simulink model "dynamic_model_tab"  (R2022b)
settings: Solver=VariableStepAuto  StartTime=0.0  StopTime=30e-2  RelTol=1e-3
undefined symbols (not defined in the file): Ion, Lithium
libraries: spsMosfetLib x12, spsMeanLib x8, eeGeneralControl x7, spsSeriesRLCBranchLib x6, spsCurrentMeasurementLib x4, spsMultimeterLib x3, slpidlib x3, hdlsllib x2, simulink x2, spsDiscreteVariableTimeDelayLib x2, spsEdgeDetectorLib x2, spsBatteryLib x1
settings Model: Creator=srikr  LastModifiedBy=srikri

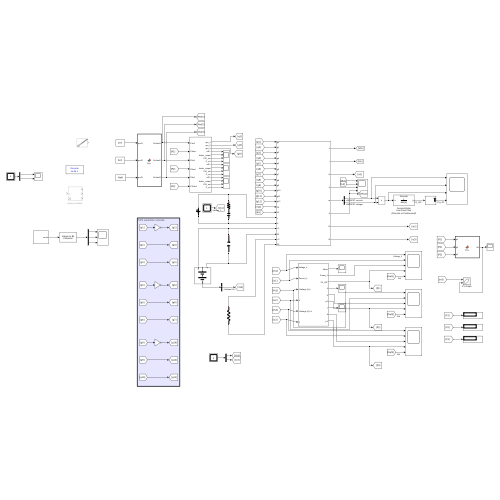
[thumbnail: Simulink's stored preview of the top-level diagram]
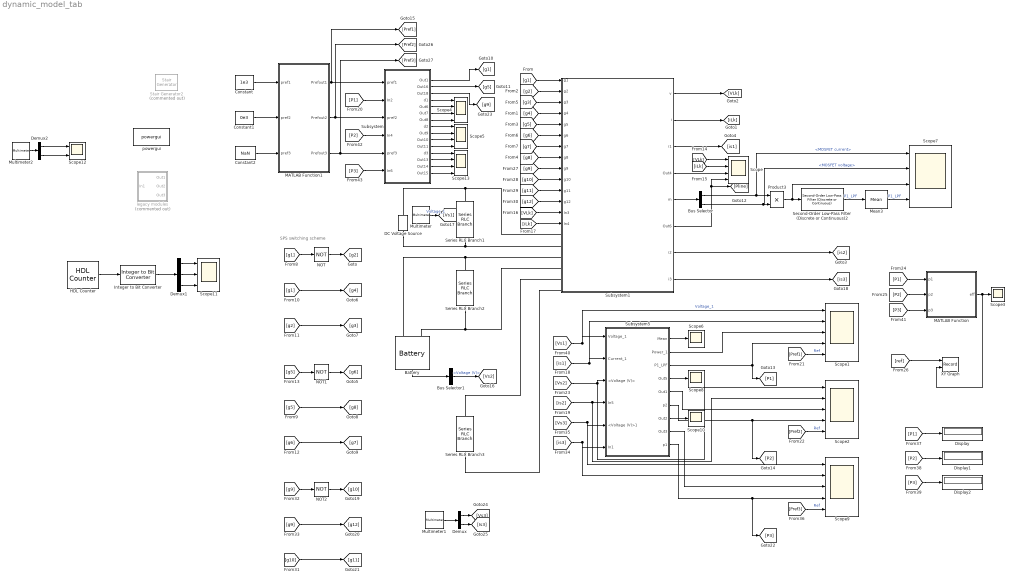
== system dynamic_model_tab ==
  note: SPS switching scheme
  Battery : spsBatteryLib/Battery  BatType=Lithium-Ion  ShowTempParam=off  ThermalPreset=no  ShowAgeParam=off  NomV=96  NomQ=150  SOC=100  Batt_Tr=30  PresetModel=on  MaxQ=150  MinV=72  FullV=111.7428  Dis_rate=65.2174  R=0.0064  Normal_OP=135.6522  expZone="[103.717      7.369565]"  current=[6.5 13 32.5]  Units=Time  Tci=20  NomT=20  T2=-30  MaxQ2=4.8  FullV2=7.1  Normal_OP2=5.655  expZone2="[6.58           1]"  Rca=0.6  ti=2000  Dp=0  Neq0=0  Tsim=1e6  Ta1=25  Qeol=5.4*0.9  Reol=0.013333*1.2  Char_age=[2.3478, 3]  Dis_age=[2.3478, 10]  N1=1500  N2=10500  N3=1000  N4=1400  Ta2=45  N5=950
  Bus Selector : BusSelector  OutputSignals=MOSFET current,MOSFET voltage
  Bus Selector1 : BusSelector  OutputSignals=Voltage (V)
  Constant : Constant  Value=1e3
  Constant1 : Constant  Value=0e3
  Constant2 : Constant  Value=NaN
  DC Voltage Source : spsDCVoltageSourceLib/DC Voltage Source  Amplitude=120  Measurements=Voltage
  Demux : Demux  Outputs=2
  Demux1 : Demux  Outputs=3
  Demux2 : Demux  Outputs=2
  Display : Display
  Display1 : Display
  Display2 : Display
  HDL Counter : hdlsllib/Sources/HDL Counter  CountType=Modulo  CountInit=0  CountStep=1  CountMax=7  CountFromType=Initial value  CountFrom=0  CountResetPort=off  CountLoadPort=off  CountEnbPort=off  CountDirPort=off  CountHitOutputPort=off  CountDataType=Unsigned  CountWordLen=8  CountFracLen=0  CountSampTime=1e-3
  Integer to Bit Converter : simulink/Logic and Bit Operations/Integer to Bit Converter  nbits=3  signedInputValues=Unsigned  bitOrder=MSB first  outDtype=Inherit via internal rule
  MATLAB Function : MATLAB Function  TreatAsAtomicUnit=on
  MATLAB Function1 : MATLAB Function  TreatAsAtomicUnit=on
  Mean3 : spsMeanLib/Mean  Freq=50e3  Vinit=0  Ts=0
  Multimeter : spsMultimeterLib/Multimeter  L=12  sel=5  yselected={}  Gain=1  OutputType=Complex  PlotAtSimulationStop=off  PhasorSimulation=off
  Multimeter1 : spsMultimeterLib/Multimeter  L=12  sel=[1 3]  yselected={}  Gain=[1 1]  OutputType=Complex  PlotAtSimulationStop=off  PhasorSimulation=off
  Multimeter2 : spsMultimeterLib/Multimeter  L=12  sel=[2 7]  yselected={}  Gain=[1 1]  OutputType=Complex  PlotAtSimulationStop=off  PhasorSimulation=off
  NOT : Logic  Operator=NOT  IconShape=distinctive  AllPortsSameDT=off  OutDataTypeStr=boolean
  NOT1 : Logic  Operator=NOT  IconShape=distinctive  AllPortsSameDT=off  OutDataTypeStr=boolean
  NOT2 : Logic  Operator=NOT  IconShape=distinctive  AllPortsSameDT=off  OutDataTypeStr=boolean
  Product3 : Product
  Scope{,4..5,7,13} (5 alike) : Scope  NumInputPorts=4
  Scope1 : Scope  NumInputPorts=5
  Scope{3,6,8,10} (4 alike) : Scope
  Scope11 : Scope  NumInputPorts=3
  Scope12 : Scope  NumInputPorts=2
  Scope2 : Scope  NumInputPorts=5
  Scope9 : Scope  NumInputPorts=5
  Second-Order Low-Pass Filter (Discrete or Continuous)2 : eeGeneralControl/Second-Order Low-Pass Filter (Discrete or Continuous)  A1=2*sqrt(2)*1e-3  A2=(1e-3)^2  init_option=Inherited from block input  x0=0  Ts=-1
      settings: LibrarySourceBlock=|
      | ee_sl_lib/General Control/Second-Order
      | Low-Pass Filter
      | (Discrete or Continuous)
  Series RLC Branch1 : spsSeriesRLCBranchLib/Series RLC Branch  LConnTagsString=__new0  RConnTagsString=__new0  BranchType=RC  Resistance=1e-9  Inductance=1e-3  SetiL0=off  InitialCurrent=0  Capacitance=1000e-6  Setx0=off  InitialVoltage=0  Measurements=None
  Series RLC Branch2 : spsSeriesRLCBranchLib/Series RLC Branch  LConnTagsString=__new0  RConnTagsString=__new0  BranchType=C  Resistance=1e-9  Inductance=1e-3  SetiL0=off  InitialCurrent=0  Capacitance=1000e-6  Setx0=off  InitialVoltage=0  Measurements=None
  Series RLC Branch3 : spsSeriesRLCBranchLib/Series RLC Branch  LConnTagsString=__new0  RConnTagsString=__new0  BranchType=R  Resistance=(380^2) / (7.5e3)  Inductance=1e-3  SetiL0=off  InitialCurrent=0  Capacitance=1000e-6  Setx0=off  InitialVoltage=0  Measurements=Branch voltage and current
  Stair Generator2 : spsStairGeneratorLib/Stair Generator  Commented=on  t=[0:0.025:1]*100e-2*(1-0.1)  e=([-1:0.05:1])*2.8e3  Ts=0
  Subsystem : Subsystem
  Subsystem1 : Subsystem
  Subsystem5 : Subsystem
  XY Graph : Record  FileSettingsInternal="{\"entries\":[{\"content\":{\"excelSettings\":{\"content\":{},\"type\":\"Streamout.ExcelSettings\"}},\"type\":\"Streamout.FileSettingStorage\",\"uuid\":\"f45d7055-9ecb-48ab-a96f-031432f1a6f8\"}],\"packageUris\":[\"http://schema.mathworks.com/mf0/streamout_blocks/R2020a\"],\"version\":\"1.0\"}"  Layout=[1 1]  SignalsInternal="{\"entries\":[{\"content\":{\"signals\":[{\"content\":{\"blockPath\":[\"dynamic_model_tab/XY Graph\"],\"channel\":[],\"dimensions\":[1],\"domain\":\"dynamic_model_tab/XY Graph\",\"lineColor\":\"#7e2f8e\",\"plots\":[],\"port\":1,\"sid\":[],\"signalID\":33,\"signalName\":\"From26\"},\"type\":\"RecordBlkView.Signal\",\"uuid\":\"0354a216-3750-4216-9fc3-88f8f814a368\"},{\"content\":{\"blockPath\":[\"dynamic_model_tab/XY Graph\"],\"channel\":[],\"dimensions\":[1],\"domain\":\"dynamic_model_tab/XY Graph\",\"lineColor\":\"#ff13a6\",\"plots\":[],\"port\":2,\"sid\":[],\"signalID\":36,\"signalName\":\"MATLAB Function\"},\"type\":\"RecordBlkView.Signal\",\"uuid\":\"1e314882-d803-43e1-8662-509fc0bc40a2\"}]},\"type\":\"RecordBlkView.InputSignals\",\"uuid\":\"ae186877-b2c7-4f81-851d-3e3b29c6325c\"}],\"packageUris\":[\"http://schema.mathworks.com/mf0/streamout_blocks/R2020a\"],\"version\":\"1.0\"}"  VisualizationBindings="{\"xyplotplugin\":{\"info\":[{\"series\":[],\"subplotID\":1}]}}"  CompatibilityTag=XY
  legacy modules : Subsystem  Commented=on
  powergui : spspowerguiLib/powergui  Priority=1  SimulationMode=Discrete  SampleTime=1e-6  frequency=60  Iterations=50  frequencyindice=0  Pbase=100e6  ErrMax=1e-4  UnitsV=kV  UnitsW=MW  buscounter=0  FunctionMessages=off  echomessages=off  EnableUseOfTLC=off  CurrentSourceSwitches=off  DisableSnubberDevices=off  DisableRonSwitches=off  DisableVfSwitches=off  DisplayEquations=off  AutomaticDiscreteSolvers=off  SolverType=Tustin/Backward Euler (TBE)  Interpol=off  ExternalGateDelay=off  methode=off  Ts=100  x0status=blocks  SPID=on  SwTol=0  HookPort=off  NonlinearTolerance=1e-4  nMaxIteration=100  ContinueOnMaxIteration=off  RestoreLinks=warning  ResistiveCurrentMeasurement=off  Frange=[0:2:500]  Ylog=off  Xlog=on  ShowGrid=off  save=off  variable=ZData  structure=0  ZoomFFT=off  StartTime=0.0  cycles=1  DisplayStyle=1  fundamental=60  FreqAxis=off  MaxFrequency=1000  frequencyindicesteady=1  RmsSteady=1  display=off
  wires:
  [VLk] -> Scope/1
  [iLk] -> Scope/2
  [Vs1] -> Scope1/1, Subsystem5/1(Voltage_1)  "Voltage_1"
  [is2] -> Subsystem5/4(In5), Scope2/2
  Bus Selector/1 -> Scope7/1, Product3/1  "<MOSFET current>"
  Bus Selector/2 -> Scope7/2, Product3/2  "<MOSFET voltage>"
  Product3/1 -> Scope7/3, Second-Order Low-Pass Filter (Discrete or Continuous)2/1
  [Pref1] -> Scope1/5  "Ref"
  Battery/1 -> Bus Selector1/1
  [P1] -> Subsystem/2(In2)
  Subsystem/1(Out1) -> [g1]
  Subsystem/2(Out16) -> [g5]
  Subsystem/4(d1) -> Scope4/1
  Subsystem/5(Out6) -> Scope4/2
  Subsystem/6(Out7) -> Scope4/3
  Subsystem/7(Out8) -> Scope4/4
  Subsystem5/1(Mean) -> Scope6/1
  Subsystem5/2(Power_1) -> Scope1/3
  Subsystem1/6(Out6) -> [Pline], Scope/4
  [g4] -> Subsystem1/4(g4)
  [g2] -> Subsystem1/2(g2)
  [VLk] -> Subsystem1/13(In3)
  [iLk] -> Subsystem1/14(In4)
  [g1] -> Subsystem1/1(g1)
  [g3] -> Subsystem1/3(g3)
  [g5] -> Subsystem1/5(g5)
  [g7] -> Subsystem1/7(g7)
  [g6] -> Subsystem1/6(g6)
  [g8] -> Subsystem1/8(g8)
  Subsystem1/1(v) -> [VLk]
  Subsystem1/2(i) -> [iLk]
  Subsystem1/3(i1) -> [is1]
  Subsystem1/4(Out4) -> Scope/3
  Subsystem1/5(m) -> Bus Selector/1
  Subsystem1/7(i2) -> [is2]
  [g1] -> NOT/1
  NOT/1 -> [g2]
  [g5] -> [g8]
  NOT1/1 -> [g6]
  [g6] -> [g7]
  [g5] -> NOT1/1
  [g2] -> [g3]
  [g1] -> [g4]
  Subsystem5/5(Out1) -> Scope2/3
  [is1] -> Scope1/2, Subsystem5/2(Current_1)
  [Pref2] -> Scope2/5  "Ref"
  Bus Selector1/1 -> [Vs2]  "<Voltage (V)>"
  [Vs2] -> Subsystem5/3(<Voltage (V)>), Scope2/1
  Second-Order Low-Pass Filter (Discrete or Continuous)2/1 -> Mean3/1  "P1_LPF"
  Mean3/1 -> Scope7/4  "P1_LPF"
  Subsystem5/3(P1_LPF) -> [P1], Scope1/4
  MATLAB Function/1(eff) -> XY Graph/2, Scope3/1
  Subsystem5/4(Out5) -> Scope8/1
  Subsystem5/6(p2) -> [P2], Scope2/4
  [P1] -> MATLAB Function/1(p1)
  [P2] -> MATLAB Function/2(p2)
  [ref] -> XY Graph/1
  [g9] -> Subsystem1/9(g9)
  [g10] -> Subsystem1/10(g10)
  [g11] -> Subsystem1/11(g11)
  [g12] -> Subsystem1/12(g12)
  Subsystem1/8(i3) -> [is3]
  [g9] -> [g12]
  [g9] -> NOT2/1
  [g10] -> [g11]
  NOT2/1 -> [g10]
  [Vs3] -> Scope9/1, Subsystem5/5(<Voltage (V)>1)
  [Pref3] -> Scope9/5  "Ref"
  [is3] -> Scope9/2, Subsystem5/6(In1)
  Subsystem5/9(p1) -> [P3], Scope9/4
  Subsystem5/8(Out3) -> Scope9/3
  Subsystem5/7(Out2) -> Scope10/1
  Subsystem/3(Out18) -> [g9]
  [P1] -> Display/1
  [P2] -> Display1/1
  [P3] -> Display2/1
  Multimeter/1 -> [Vs1]  "Voltage_1"
  Multimeter1/1 -> Demux/1
  Demux/1 -> [Vs3]
  Demux/2 -> [Is3]
  Integer to Bit Converter/1 -> Demux1/1
  HDL Counter/1 -> Integer to Bit Converter/1
  Demux1/1 -> Scope11/1
  Demux1/2 -> Scope11/2
  Demux1/3 -> Scope11/3
  Multimeter2/1 -> Demux2/1
  Demux2/1 -> Scope12/1
  Demux2/2 -> Scope12/2
  [P3] -> MATLAB Function/3(p3)
  Subsystem/11(Out11) -> Scope5/4
  Subsystem/9(Out9) -> Scope5/2
  Subsystem/8(d2) -> Scope5/1
  Subsystem/10(Out10) -> Scope5/3
  Subsystem/15(Out15) -> Scope13/4
  Subsystem/13(Out13) -> Scope13/2
  Subsystem/12(d3) -> Scope13/1
  Subsystem/14(Out14) -> Scope13/3
  [P2] -> Subsystem/4(In4)
  [P3] -> Subsystem/6(In6)
  Constant/1 -> MATLAB Function1/1(pref1)
  Constant1/1 -> MATLAB Function1/2(pref2)
  Constant2/1 -> MATLAB Function1/3(pref3)
  MATLAB Function1/1(Prefout1) -> Subsystem/1(pref1), [Pref1]
  MATLAB Function1/2(Prefout2) -> Subsystem/3(pref2), [Pref2]
  MATLAB Function1/3(Prefout3) -> Subsystem/5(pref3), [Pref3]
  connections:
  Series RLC Branch1/RConn1 -- DC Voltage Source/LConn1 -- Subsystem1/LConn2
  Series RLC Branch2/RConn1 -- Subsystem1/LConn4 -- Battery/LConn2
  Series RLC Branch2/LConn1 -- Subsystem1/LConn3 -- Battery/LConn1
  Subsystem1/LConn1 -- DC Voltage Source/RConn1 -- Series RLC Branch1/LConn1
  Series RLC Branch3/RConn1 -- Subsystem1/LConn6
  Series RLC Branch3/LConn1 -- Subsystem1/LConn5

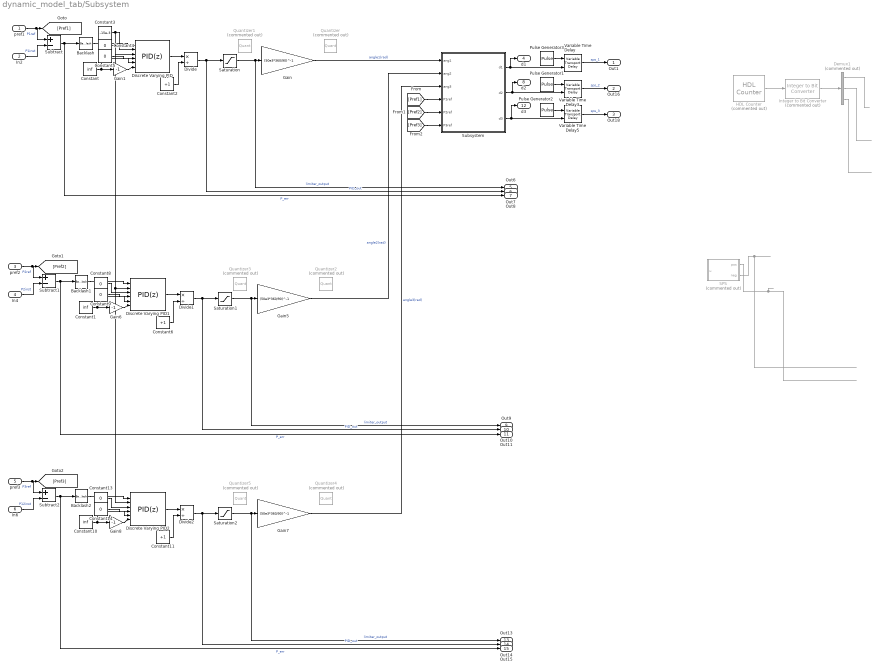
== system dynamic_model_tab/Subsystem ==
  pref1 : Inport
  In2 : Inport  Port=2
  pref2 : Inport  Port=3
  In4 : Inport  Port=4
  pref3 : Inport  Port=5
  In6 : Inport  Port=6
  Backlash : Backlash  BacklashWidth=0
  Backlash1 : Backlash  BacklashWidth=0
  Backlash2 : Backlash  BacklashWidth=0
  Constant : Constant  Value=inf
  Constant1 : Constant  Value=inf
  Constant10 : Constant  Value=inf
  Constant11 : Constant  Value=+1
  Constant{4..5,8..9,13..14} (6 alike) : Constant  Value=0
  Constant2 : Constant  Value=+1
  Constant3 : Constant  Value=-15e-3
  Constant6 : Constant  Value=+1
  Demux1 : Demux  Commented=on  Outputs=3
  Discrete Varying PID : slpidlib/PID Controller  Controller=PID  Form=Parallel  TimeDomain=Discrete-time  UseExternalTs=off  SampleTime=-1  IntegratorMethod=Forward Euler  FilterMethod=Forward Euler  ControllerParametersSource=external  P=1  I=1  UseKiTs=off  D=0  N=100  UseFilter=off  TunerSelectOption=Transfer Function Based (PID Tuner App)  InitialConditionSource=internal  InitialConditionForIntegrator=0  InitialConditionForFilter=0  DifferentiatorICPrevScaledInput=0  ExternalReset=none  TrackingMode=off  Kt=1  LimitOutput=on  SatLimitsSource=external  UpperSaturationLimit=inf  LowerSaturationLimit=-inf  LinearizeAsGain=on  AntiWindupMode=none  Kb=1  LimitIntegrator=off  UpperIntegratorSaturationLimit=inf  LowerIntegratorSaturationLimit=-inf  POutMin=[]  POutMax=[]  IOutMin=[]  IOutMax=[]  DOutMin=[]  DOutMax=[]  NOutMin=[]  NOutMax=[]  SumOutMin=[]  SumOutMax=[]  SaturationOutMin=[]  SaturationOutMax=[]  PParamMin=[]  PParamMax=[]  IParamMin=[]  IParamMax=[]  DParamMin=[]  DParamMax=[]  NParamMin=[]  NParamMax=[]  KbParamMin=[]  KbParamMax=[]  KtParamMin=[]  KtParamMax=[]  KbOutMin=[]  KbOutMax=[]  KtOutMin=[]  KtOutMax=[]  IntegratorOutMin=[]  IntegratorOutMax=[]  FilterOutMin=[]  FilterOutMax=[]  SumI1OutMin=[]  SumI1OutMax=[]  SumI2OutMin=[]  SumI2OutMax=[]  SumI3OutMin=[]  SumI3OutMax=[]  SumI4OutMin=[]  SumI4OutMax=[]  SumDOutMin=[]  SumDOutMax=[]  DifferentiatorOutMin=[]  DifferentiatorOutMax=[]  FilterDiffOutCoefMin=[]  FilterDiffOutCoefMax=[]  ReciprocalOutMin=[]  ReciprocalOutMax=[]  SumDenOutMin=[]  SumDenOutMax=[]  SumNumOutMin=[]  SumNumOutMax=[]  DivideOutMin=[]  DivideOutMax=[]  UdiffTsProdOutMin=[]  UdiffTsProdOutMax=[]  NTsProdOutMin=[]  NTsProdOutMax=[]  UintegralTsProdOutMin=[]  UintegralTsProdOutMax=[]  UngainTsProdOutMin=[]  UngainTsProdOutMax=[]  ClampingZeroOutDataTypeStr=Inherit: Inherit via back propagation  ClampingZeroOutMin=[]  ClampingZeroOutMax=[]  FilterDenConstantOutDataTypeStr=Inherit: Inherit via back propagation  FilterDenConstantOutMin=[]  FilterDenConstantOutMax=[]  PCopyOutDataTypeStr=Inherit: Inherit via back propagation  PCopyOutMin=[]  PCopyOutMax=[]  NCopyOutDataTypeStr=Inherit: Inherit via back propagation  NCopyOutMin=[]  NCopyOutMax=[]  IntegratorContinuousStateAttributes=''  IntegratorStateMustResolveToSignalObject=off  IntegratorRTWStateStorageClass=Auto  FilterContinuousStateAttributes=''  FilterStateMustResolveToSignalObject=off  FilterRTWStateStorageClass=Auto  ParallelPVariant=ExternalParameters  IdealPVariant=Disabled  IVariant=ExternalParameters  DVariant=ExternalParameters  IntegratorVariant=Discrete  SatVariant=External  AWVariant=Passthrough  PCopyVariant=Disabled  TRVariant=Disabled  FdbkBlocksVariant=Forward  IdealPFdbkVariant=Disabled  SatFdbkVariant=Disabled  DerivativeFilterVariant=Differentiator  NVariant=Passthrough  NCopyVariant=Disabled_SignalSpec  FilterICVariant=InternalICsDifferentiator  IntegratorICVariant=InternalICs  ExternalResetVariant=Disabled  TRSumVariant=Passthrough  SumFdbkVariant=Disabled  SumVariant=Sum_PID  TsampFilterVariant=InternalTs  TsampNgainVariant=Passthrough  TsampIntegralVariant=Passthrough  ExternalSaturationOutDataTypeStr=Inherit: Same as second input
      settings: LibrarySourceBlock=cstblocks/Linear Parameter Varying/Discrete Varying PID
  Discrete Varying PID1 : slpidlib/PID Controller  Controller=PID  Form=Parallel  TimeDomain=Discrete-time  UseExternalTs=off  SampleTime=-1  IntegratorMethod=Forward Euler  FilterMethod=Forward Euler  ControllerParametersSource=external  P=1  I=1  UseKiTs=off  D=0  N=100  UseFilter=off  TunerSelectOption=Transfer Function Based (PID Tuner App)  InitialConditionSource=internal  InitialConditionForIntegrator=0  InitialConditionForFilter=0  DifferentiatorICPrevScaledInput=0  ExternalReset=none  TrackingMode=off  Kt=1  LimitOutput=on  SatLimitsSource=external  UpperSaturationLimit=inf  LowerSaturationLimit=-inf  LinearizeAsGain=on  AntiWindupMode=none  Kb=1  LimitIntegrator=off  UpperIntegratorSaturationLimit=inf  LowerIntegratorSaturationLimit=-inf  POutMin=[]  POutMax=[]  IOutMin=[]  IOutMax=[]  DOutMin=[]  DOutMax=[]  NOutMin=[]  NOutMax=[]  SumOutMin=[]  SumOutMax=[]  SaturationOutMin=[]  SaturationOutMax=[]  PParamMin=[]  PParamMax=[]  IParamMin=[]  IParamMax=[]  DParamMin=[]  DParamMax=[]  NParamMin=[]  NParamMax=[]  KbParamMin=[]  KbParamMax=[]  KtParamMin=[]  KtParamMax=[]  KbOutMin=[]  KbOutMax=[]  KtOutMin=[]  KtOutMax=[]  IntegratorOutMin=[]  IntegratorOutMax=[]  FilterOutMin=[]  FilterOutMax=[]  SumI1OutMin=[]  SumI1OutMax=[]  SumI2OutMin=[]  SumI2OutMax=[]  SumI3OutMin=[]  SumI3OutMax=[]  SumI4OutMin=[]  SumI4OutMax=[]  SumDOutMin=[]  SumDOutMax=[]  DifferentiatorOutMin=[]  DifferentiatorOutMax=[]  FilterDiffOutCoefMin=[]  FilterDiffOutCoefMax=[]  ReciprocalOutMin=[]  ReciprocalOutMax=[]  SumDenOutMin=[]  SumDenOutMax=[]  SumNumOutMin=[]  SumNumOutMax=[]  DivideOutMin=[]  DivideOutMax=[]  UdiffTsProdOutMin=[]  UdiffTsProdOutMax=[]  NTsProdOutMin=[]  NTsProdOutMax=[]  UintegralTsProdOutMin=[]  UintegralTsProdOutMax=[]  UngainTsProdOutMin=[]  UngainTsProdOutMax=[]  ClampingZeroOutDataTypeStr=Inherit: Inherit via back propagation  ClampingZeroOutMin=[]  ClampingZeroOutMax=[]  FilterDenConstantOutDataTypeStr=Inherit: Inherit via back propagation  FilterDenConstantOutMin=[]  FilterDenConstantOutMax=[]  PCopyOutDataTypeStr=Inherit: Inherit via back propagation  PCopyOutMin=[]  PCopyOutMax=[]  NCopyOutDataTypeStr=Inherit: Inherit via back propagation  NCopyOutMin=[]  NCopyOutMax=[]  IntegratorContinuousStateAttributes=''  IntegratorStateMustResolveToSignalObject=off  IntegratorRTWStateStorageClass=Auto  FilterContinuousStateAttributes=''  FilterStateMustResolveToSignalObject=off  FilterRTWStateStorageClass=Auto  ParallelPVariant=ExternalParameters  IdealPVariant=Disabled  IVariant=ExternalParameters  DVariant=ExternalParameters  IntegratorVariant=Discrete  SatVariant=External  AWVariant=Passthrough  PCopyVariant=Disabled  TRVariant=Disabled  FdbkBlocksVariant=Forward  IdealPFdbkVariant=Disabled  SatFdbkVariant=Disabled  DerivativeFilterVariant=Differentiator  NVariant=Passthrough  NCopyVariant=Disabled_SignalSpec  FilterICVariant=InternalICsDifferentiator  IntegratorICVariant=InternalICs  ExternalResetVariant=Disabled  TRSumVariant=Passthrough  SumFdbkVariant=Disabled  SumVariant=Sum_PID  TsampFilterVariant=InternalTs  TsampNgainVariant=Passthrough  TsampIntegralVariant=Passthrough  ExternalSaturationOutDataTypeStr=Inherit: Same as second input
      settings: LibrarySourceBlock=cstblocks/Linear Parameter Varying/Discrete Varying PID
  Discrete Varying PID2 : slpidlib/PID Controller  Controller=PID  Form=Parallel  TimeDomain=Discrete-time  UseExternalTs=off  SampleTime=-1  IntegratorMethod=Forward Euler  FilterMethod=Forward Euler  ControllerParametersSource=external  P=1  I=1  UseKiTs=off  D=0  N=100  UseFilter=off  TunerSelectOption=Transfer Function Based (PID Tuner App)  InitialConditionSource=internal  InitialConditionForIntegrator=0  InitialConditionForFilter=0  DifferentiatorICPrevScaledInput=0  ExternalReset=none  TrackingMode=off  Kt=1  LimitOutput=on  SatLimitsSource=external  UpperSaturationLimit=inf  LowerSaturationLimit=-inf  LinearizeAsGain=on  AntiWindupMode=none  Kb=1  LimitIntegrator=off  UpperIntegratorSaturationLimit=inf  LowerIntegratorSaturationLimit=-inf  POutMin=[]  POutMax=[]  IOutMin=[]  IOutMax=[]  DOutMin=[]  DOutMax=[]  NOutMin=[]  NOutMax=[]  SumOutMin=[]  SumOutMax=[]  SaturationOutMin=[]  SaturationOutMax=[]  PParamMin=[]  PParamMax=[]  IParamMin=[]  IParamMax=[]  DParamMin=[]  DParamMax=[]  NParamMin=[]  NParamMax=[]  KbParamMin=[]  KbParamMax=[]  KtParamMin=[]  KtParamMax=[]  KbOutMin=[]  KbOutMax=[]  KtOutMin=[]  KtOutMax=[]  IntegratorOutMin=[]  IntegratorOutMax=[]  FilterOutMin=[]  FilterOutMax=[]  SumI1OutMin=[]  SumI1OutMax=[]  SumI2OutMin=[]  SumI2OutMax=[]  SumI3OutMin=[]  SumI3OutMax=[]  SumI4OutMin=[]  SumI4OutMax=[]  SumDOutMin=[]  SumDOutMax=[]  DifferentiatorOutMin=[]  DifferentiatorOutMax=[]  FilterDiffOutCoefMin=[]  FilterDiffOutCoefMax=[]  ReciprocalOutMin=[]  ReciprocalOutMax=[]  SumDenOutMin=[]  SumDenOutMax=[]  SumNumOutMin=[]  SumNumOutMax=[]  DivideOutMin=[]  DivideOutMax=[]  UdiffTsProdOutMin=[]  UdiffTsProdOutMax=[]  NTsProdOutMin=[]  NTsProdOutMax=[]  UintegralTsProdOutMin=[]  UintegralTsProdOutMax=[]  UngainTsProdOutMin=[]  UngainTsProdOutMax=[]  ClampingZeroOutDataTypeStr=Inherit: Inherit via back propagation  ClampingZeroOutMin=[]  ClampingZeroOutMax=[]  FilterDenConstantOutDataTypeStr=Inherit: Inherit via back propagation  FilterDenConstantOutMin=[]  FilterDenConstantOutMax=[]  PCopyOutDataTypeStr=Inherit: Inherit via back propagation  PCopyOutMin=[]  PCopyOutMax=[]  NCopyOutDataTypeStr=Inherit: Inherit via back propagation  NCopyOutMin=[]  NCopyOutMax=[]  IntegratorContinuousStateAttributes=''  IntegratorStateMustResolveToSignalObject=off  IntegratorRTWStateStorageClass=Auto  FilterContinuousStateAttributes=''  FilterStateMustResolveToSignalObject=off  FilterRTWStateStorageClass=Auto  ParallelPVariant=ExternalParameters  IdealPVariant=Disabled  IVariant=ExternalParameters  DVariant=ExternalParameters  IntegratorVariant=Discrete  SatVariant=External  AWVariant=Passthrough  PCopyVariant=Disabled  TRVariant=Disabled  FdbkBlocksVariant=Forward  IdealPFdbkVariant=Disabled  SatFdbkVariant=Disabled  DerivativeFilterVariant=Differentiator  NVariant=Passthrough  NCopyVariant=Disabled_SignalSpec  FilterICVariant=InternalICsDifferentiator  IntegratorICVariant=InternalICs  ExternalResetVariant=Disabled  TRSumVariant=Passthrough  SumFdbkVariant=Disabled  SumVariant=Sum_PID  TsampFilterVariant=InternalTs  TsampNgainVariant=Passthrough  TsampIntegralVariant=Passthrough  ExternalSaturationOutDataTypeStr=Inherit: Same as second input
      settings: LibrarySourceBlock=cstblocks/Linear Parameter Varying/Discrete Varying PID
  Divide : Product  Inputs=*/
  Divide1 : Product  Inputs=*/
  Divide2 : Product  Inputs=*/
  Gain : Gain  Gain=(50e3*360/90)^-1
  Gain1 : Gain  Gain=-1
  Gain5 : Gain  Gain=(50e3*360/90)^-1
  Gain6 : Gain  Gain=-1
  Gain7 : Gain  Gain=(50e3*360/90)^-1
  Gain8 : Gain  Gain=-1
  HDL Counter : hdlsllib/Sources/HDL Counter  Commented=on  CountType=Modulo  CountInit=0  CountStep=1  CountMax=7  CountFromType=Initial value  CountFrom=0  CountResetPort=off  CountLoadPort=off  CountEnbPort=off  CountDirPort=off  CountHitOutputPort=off  CountDataType=Unsigned  CountWordLen=8  CountFracLen=0  CountSampTime=3e-2
  Integer to Bit Converter : simulink/Logic and Bit Operations/Integer to Bit Converter  Commented=on  nbits=3  signedInputValues=Unsigned  bitOrder=MSB first  outDtype=double
  Pulse Generator1 : DiscretePulseGenerator  PulseType=Time based  Period=1/50e3  PulseWidth=50
  Pulse Generator2 : DiscretePulseGenerator  PulseType=Time based  Period=1/50e3  PulseWidth=50
  Pulse Generator3 : DiscretePulseGenerator  PulseType=Time based  Period=1/50e3  PulseWidth=50
  Quantizer : Quantizer  Commented=on  QuantizationInterval=1e-5
  Quantizer1 : Quantizer  Commented=on  QuantizationInterval=1e-2
  Quantizer2 : Quantizer  Commented=on  QuantizationInterval=1e-5
  Quantizer3 : Quantizer  Commented=on  QuantizationInterval=1e-2
  Quantizer4 : Quantizer  Commented=on  QuantizationInterval=1e-5
  Quantizer5 : Quantizer  Commented=on  QuantizationInterval=1e-2
  SPS : MATLAB Function  Commented=on  TreatAsAtomicUnit=on
  Saturation : Saturate  UpperLimit=1  LowerLimit=0
  Saturation1 : Saturate  UpperLimit=1  LowerLimit=0
  Saturation2 : Saturate  UpperLimit=1  LowerLimit=0
  Subsystem : Subsystem
  Subtract : Sum  Inputs=+-
  Subtract1 : Sum  Inputs=+-
  Subtract2 : Sum  Inputs=+-
  Variable Time Delay : VariableTransportDelay  MaximumDelay=10
  Variable Time Delay3 : VariableTransportDelay  MaximumDelay=10
  Variable Time Delay5 : VariableTransportDelay  MaximumDelay=10
  Out1 : Outport
  Out16 : Outport  Port=2
  Out18 : Outport  Port=3
  d1 : Outport  Port=4
  Out6 : Outport  Port=5
  Out7 : Outport  Port=6
  Out8 : Outport  Port=7
  d2 : Outport  Port=8
  Out9 : Outport  Port=9
  Out10 : Outport  Port=10
  Out11 : Outport  Port=11
  d3 : Outport  Port=12
  Out13 : Outport  Port=13
  Out14 : Outport  Port=14
  Out15 : Outport  Port=15
  wires:
  Backlash/1 -> Discrete Varying PID/1
  Constant2/1 -> Divide/2
  Constant4/1 -> Discrete Varying PID/3
  pref1/1 -> Subtract/1, [Pref1]  "P1ref"
  Variable Time Delay/1 -> Out1/1  "sps_1"
  Saturation/1 -> Out6/1, Gain/1  "limiter_output"
  In2/1 -> Subtract/2  "P1inst"
  Constant/1 -> Discrete Varying PID/5, Gain1/1
  Constant5/1 -> Discrete Varying PID/4
  Divide/1 -> Saturation/1, Out7/1  "PID_out"
  Discrete Varying PID/1 -> Divide/1
  Subtract/1 -> Out8/1, Backlash/1  "P_err"
  Gain1/1 -> Discrete Varying PID/6
  Gain/1 -> Subsystem/1(ang1)  "angle1(rad)"
  In4/1 -> Subtract1/2  "P2inst"
  Backlash1/1 -> Discrete Varying PID1/1
  Constant1/1 -> Discrete Varying PID1/5, Gain6/1
  Saturation1/1 -> Out9/1, Gain5/1  "limiter_output"
  Gain5/1 -> Subsystem/2(ang2)  "angle2(rad)"
  Constant9/1 -> Discrete Varying PID1/4
  pref2/1 -> Subtract1/1, [Pref2]  "P2ref"
  Gain6/1 -> Discrete Varying PID1/6
  Subtract1/1 -> Out11/1, Backlash1/1  "P_err"
  Discrete Varying PID1/1 -> Divide1/1
  Constant8/1 -> Discrete Varying PID1/3
  Constant6/1 -> Divide1/2
  Divide1/1 -> Saturation1/1, Out10/1  "PID_out"
  pref3/1 -> Subtract2/1, [Pref3]  "P3ref"
  Constant14/1 -> Discrete Varying PID2/4
  Gain7/1 -> Subsystem/3(ang3)  "angle3(rad)"
  Backlash2/1 -> Discrete Varying PID2/1
  Constant13/1 -> Discrete Varying PID2/3
  Saturation2/1 -> Out13/1, Gain7/1  "limiter_output"
  Constant10/1 -> Discrete Varying PID2/5, Gain8/1
  In6/1 -> Subtract2/2  "P12inst"
  Gain8/1 -> Discrete Varying PID2/6
  Constant3/1 -> Discrete Varying PID/2, Discrete Varying PID2/2, Discrete Varying PID1/2
  Subtract2/1 -> Out15/1, Backlash2/1  "P_err"
  Discrete Varying PID2/1 -> Divide2/1
  Constant11/1 -> Divide2/2
  Divide2/1 -> Saturation2/1, Out14/1  "PID_out"
  Pulse Generator1/1 -> Variable Time Delay3/1
  Variable Time Delay3/1 -> Out16/1  "sps_2"
  Variable Time Delay5/1 -> Out18/1  "sps_3"
  Pulse Generator2/1 -> Variable Time Delay5/1
  SPS/1(pos) -> ?
  SPS/2(neg) -> ?
  Demux1/1 -> ?
  Integer to Bit Converter/1 -> Demux1/1
  Demux1/3 -> ?
  Demux1/2 -> ?
  HDL Counter/1 -> Integer to Bit Converter/1
  Pulse Generator3/1 -> Variable Time Delay/1
  Subsystem/1(d1) -> d1/1, Variable Time Delay/2
  Subsystem/2(d2) -> d2/1, Variable Time Delay3/2
  Subsystem/3(d3) -> d3/1, Variable Time Delay5/2
  [Pref1] -> Subsystem/4(P1ref)
  [Pref2] -> Subsystem/5(P2ref)
  [Pref3] -> Subsystem/6(P3ref)

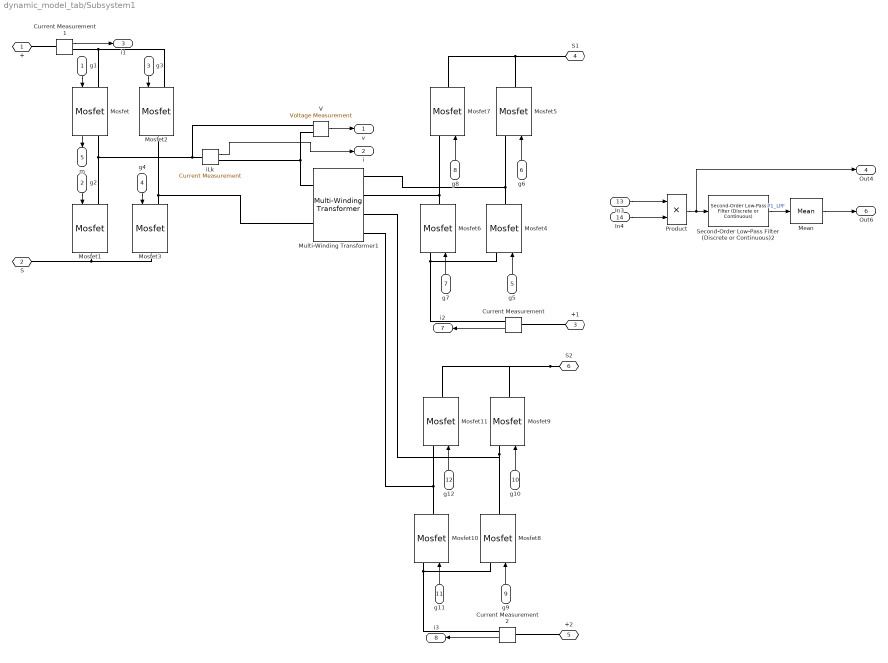
== system dynamic_model_tab/Subsystem1 ==
  g1 : Inport
  g2 : Inport  Port=2
  g3 : Inport  Port=3
  g4 : Inport  Port=4
  g5 : Inport  Port=5
  g6 : Inport  Port=6
  g7 : Inport  Port=7
  g8 : Inport  Port=8
  g9 : Inport  Port=9
  g10 : Inport  Port=10
  g11 : Inport  Port=11
  g12 : Inport  Port=12
  In3 : Inport  Port=13
  In4 : Inport  Port=14
  Current Measurement : spsCurrentMeasurementLib/Current Measurement  PhasorSimulation=off  OutputType=Complex  PSBequivalent=0
  Current Measurement1 : spsCurrentMeasurementLib/Current Measurement  PhasorSimulation=off  OutputType=Complex  PSBequivalent=0
  Current Measurement2 : spsCurrentMeasurementLib/Current Measurement  PhasorSimulation=off  OutputType=Complex  PSBequivalent=0
  Mean : spsMeanLib/Mean  Freq=50e3  Vinit=0  Ts=0
  Mosfet : spsMosfetLib/Mosfet  Ron=0.1  Lon=0  Rd=0.01  Vfd=0  IC=0  Rs=1e6  Cs=inf  Measurements=on
  Mosfet1 : spsMosfetLib/Mosfet  Ron=0.1  Lon=0  Rd=0.01  Vfd=0  IC=0  Rs=inf  Cs=inf  Measurements=off
  Mosfet{2..11} (10 alike) : spsMosfetLib/Mosfet  Ron=0.1  Lon=0  Rd=0.01  Vfd=0  IC=0  Rs=1e6  Cs=inf  Measurements=off
  Multi-Winding Transformer1 : spsMultiWindingTransformerLib/Multi-Winding Transformer  LeftWindings=1  RightWindings=2  TappedWindings=no taps  NumberOfTaps=2  SetSaturation=off  Hysteresis=off  DataFile='hysteresis.mat'  Measurements=All measurements (V I Flux)  UNITS=SI  NominalPower=[10e3 50e3]  NominalVoltages="[ 120  96  380 ]"  WindingResistances=[ 0 0 0 ]  WindingInductances=[ 14e-6 6e-6 12.9e-6 ]  Rm=10e6  Lm=2e-3  Saturation=[0 0;0.017678 64.823;7.3657 82.109]  SpecifyInitialFlux=off  InitialFlux=0  BreakLoop=off  DiscreteSolver=Trapezoidal iterative  DataType=on  TransfoNumber=1
      settings: LibrarySourceBlock=|
      | sps_lib/Power Grid Elements/Multi-Winding
      | Transformer
  Product : Product
  Second-Order Low-Pass Filter (Discrete or Continuous)2 : eeGeneralControl/Second-Order Low-Pass Filter (Discrete or Continuous)  A1=2*sqrt(2)*1e-3  A2=(1e-3)^2  init_option=Inherited from block input  x0=0  Ts=-1
      settings: LibrarySourceBlock=|
      | ee_sl_lib/General Control/Second-Order
      | Low-Pass Filter
      | (Discrete or Continuous)
  V : spsVoltageMeasurementLib/Voltage Measurement  PhasorSimulation=off  OutputType=Complex  PSBequivalent=0
  iLk : spsCurrentMeasurementLib/Current Measurement  PhasorSimulation=off  OutputType=Complex  PSBequivalent=0
  + : PMIOPort  Side=Left
  S : PMIOPort  Port=2  Side=Left
  +1 : PMIOPort  Port=3  Side=Left
  S1 : PMIOPort  Port=4  Side=Left
  +2 : PMIOPort  Port=5  Side=Left
  S2 : PMIOPort  Port=6  Side=Left
  v : Outport
  i : Outport  Port=2
  i1 : Outport  Port=3
  Out4 : Outport  Port=4
  m : Outport  Port=5
  Out6 : Outport  Port=6
  i2 : Outport  Port=7
  i3 : Outport  Port=8
  wires:
  V/1 -> v/1
  g7/1 -> Mosfet6/1
  In3/1 -> Product/1
  g6/1 -> Mosfet5/1
  In4/1 -> Product/2
  Mosfet/1 -> m/1
  g1/1 -> Mosfet/1
  g5/1 -> Mosfet4/1
  iLk/1 -> i/1
  Current Measurement1/1 -> i1/1
  Current Measurement/1 -> i2/1
  g2/1 -> Mosfet1/1
  g4/1 -> Mosfet3/1
  Mean/1 -> Out6/1
  g3/1 -> Mosfet2/1
  g8/1 -> Mosfet7/1
  Product/1 -> Out4/1, Second-Order Low-Pass Filter (Discrete or Continuous)2/1
  Second-Order Low-Pass Filter (Discrete or Continuous)2/1 -> Mean/1  "P1_LPF"
  g11/1 -> Mosfet10/1
  g9/1 -> Mosfet8/1
  Current Measurement2/1 -> i3/1
  g12/1 -> Mosfet11/1
  g10/1 -> Mosfet9/1
  connections:
  Current Measurement1/RConn1 -- Mosfet/LConn1 -- Mosfet2/LConn1
  Current Measurement/LConn1 -- +1/RConn1
  Current Measurement/RConn1 -- Mosfet4/LConn1 -- Mosfet6/LConn1
  Current Measurement1/LConn1 -- +/RConn1
  Mosfet3/RConn1 -- S/RConn1 -- Mosfet1/RConn1
  iLk/LConn1 -- V/LConn1 -- Mosfet/RConn1 -- Mosfet1/LConn1
  V/LConn2 -- Multi-Winding Transformer1/LConn1 -- iLk/RConn1
  Mosfet7/RConn1 -- Mosfet5/RConn1 -- S1/RConn1
  Mosfet3/LConn1 -- Multi-Winding Transformer1/LConn2 -- Mosfet2/RConn1
  Mosfet4/RConn1 -- Mosfet5/LConn1 -- Multi-Winding Transformer1/RConn1
  Mosfet7/LConn1 -- Multi-Winding Transformer1/RConn2 -- Mosfet6/RConn1
  S2/RConn1 -- Mosfet11/RConn1 -- Mosfet9/RConn1
  Mosfet10/LConn1 -- Current Measurement2/RConn1 -- Mosfet8/LConn1
  Mosfet11/LConn1 -- Multi-Winding Transformer1/RConn4 -- Mosfet10/RConn1
  Mosfet9/LConn1 -- Multi-Winding Transformer1/RConn3 -- Mosfet8/RConn1
  Current Measurement2/LConn1 -- +2/RConn1

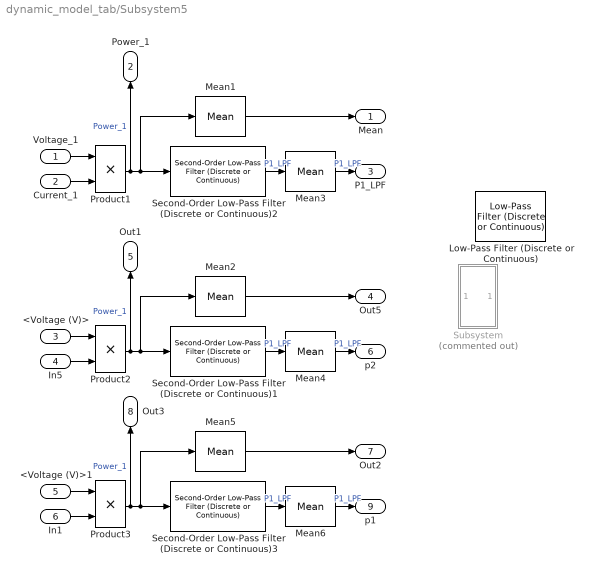
== system dynamic_model_tab/Subsystem5 ==
  Voltage_1 : Inport
  Current_1 : Inport  Port=2
  <Voltage (V)> : Inport  Port=3
  In5 : Inport  Port=4
  <Voltage (V)>1 : Inport  Port=5
  In1 : Inport  Port=6
  Low-Pass Filter (Discrete or Continuous) : eeGeneralControl/Low-Pass Filter (Discrete or Continuous)  K=1  T=1e-3  B=inf  A=-inf  init_option=Specify as parameter  x0=0  Ts=-1
  Mean{1..6} (6 alike) : spsMeanLib/Mean  Freq=50e3  Vinit=0  Ts=0
  Product1 : Product
  Product2 : Product
  Product3 : Product
  Second-Order Low-Pass Filter (Discrete or Continuous)1 : eeGeneralControl/Second-Order Low-Pass Filter (Discrete or Continuous)  A1=2*sqrt(2)*1e-3  A2=(1e-3)^2  init_option=Inherited from block input  x0=0  Ts=-1
      settings: LibrarySourceBlock=|
      | ee_sl_lib/General Control/Second-Order
      | Low-Pass Filter
      | (Discrete or Continuous)
  Second-Order Low-Pass Filter (Discrete or Continuous)2 : eeGeneralControl/Second-Order Low-Pass Filter (Discrete or Continuous)  A1=2*sqrt(2)*1e-3  A2=(1e-3)^2  init_option=Inherited from block input  x0=0  Ts=-1
      settings: LibrarySourceBlock=|
      | ee_sl_lib/General Control/Second-Order
      | Low-Pass Filter
      | (Discrete or Continuous)
  Second-Order Low-Pass Filter (Discrete or Continuous)3 : eeGeneralControl/Second-Order Low-Pass Filter (Discrete or Continuous)  A1=2*sqrt(2)*1e-3  A2=(1e-3)^2  init_option=Inherited from block input  x0=0  Ts=-1
      settings: LibrarySourceBlock=|
      | ee_sl_lib/General Control/Second-Order
      | Low-Pass Filter
      | (Discrete or Continuous)
  Subsystem : Subsystem  Commented=on
  Mean : Outport
  Power_1 : Outport  Port=2
  P1_LPF : Outport  Port=3
  Out5 : Outport  Port=4
  Out1 : Outport  Port=5
  p2 : Outport  Port=6
  Out2 : Outport  Port=7
  Out3 : Outport  Port=8
  p1 : Outport  Port=9
  wires:
  Current_1/1 -> Product1/2
  Mean1/1 -> Mean/1
  Product1/1 -> Mean1/1, Second-Order Low-Pass Filter (Discrete or Continuous)2/1, Power_1/1  "Power_1"
  <Voltage (V)>/1 -> Product2/1
  Voltage_1/1 -> Product1/1
  In5/1 -> Product2/2
  Mean2/1 -> Out5/1
  Mean3/1 -> P1_LPF/1  "P1_LPF"
  Second-Order Low-Pass Filter (Discrete or Continuous)1/1 -> Mean4/1  "P1_LPF"
  Product2/1 -> Mean2/1, Second-Order Low-Pass Filter (Discrete or Continuous)1/1, Out1/1  "Power_1"
  Mean4/1 -> p2/1  "P1_LPF"
  Second-Order Low-Pass Filter (Discrete or Continuous)2/1 -> Mean3/1  "P1_LPF"
  Mean6/1 -> p1/1  "P1_LPF"
  Mean5/1 -> Out2/1
  Product3/1 -> Out3/1, Second-Order Low-Pass Filter (Discrete or Continuous)3/1, Mean5/1  "Power_1"
  <Voltage (V)>1/1 -> Product3/1
  In1/1 -> Product3/2
  Second-Order Low-Pass Filter (Discrete or Continuous)3/1 -> Mean6/1  "P1_LPF"

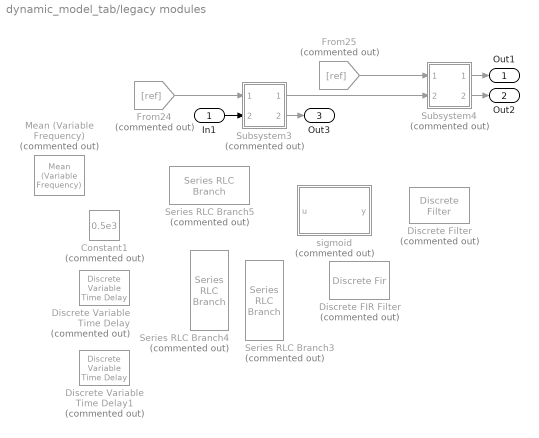
== system dynamic_model_tab/legacy modules ==
  In1 : Inport
  Constant1 : Constant  Commented=on  Value=0.5e3
  Discrete FIR Filter : DiscreteFir  Commented=on
  Discrete Filter : DiscreteFilter  Commented=on
  Discrete Variable Time Delay : spsDiscreteVariableTimeDelayLib/Discrete Variable Time Delay  Commented=on  MaxDelay=1  InitialValue=0  Ts=1e-4  DFT=on
      settings: LibrarySourceBlock=|
      | sps_lib/Control/Discrete Variable
      | Time Delay
  Discrete Variable Time Delay1 : spsDiscreteVariableTimeDelayLib/Discrete Variable Time Delay  Commented=on  MaxDelay=1  InitialValue=0  Ts=1e-4  DFT=on
      settings: LibrarySourceBlock=|
      | sps_lib/Control/Discrete Variable
      | Time Delay
  From24 : From  Commented=on  GotoTag=ref
  From25 : From  Commented=on  GotoTag=ref
  Mean (Variable Frequency) : spsMeanVariableFrequencyLib/Mean (Variable Frequency)  Commented=on  Finit=60  Fmin=45  Vinit=0  Ts=0
      settings: LibrarySourceBlock=|
      | sps_lib/Sensors and Measurements/Mean
      | (Variable Frequency)
  Series RLC Branch3 : spsSeriesRLCBranchLib/Series RLC Branch  Commented=on  LConnTagsString=__new0  RConnTagsString=__new0  BranchType=L  Resistance=1  Inductance=1e-6/(1.25^2)  SetiL0=off  InitialCurrent=0  Capacitance=1e-6  Setx0=off  InitialVoltage=0  Measurements=Branch voltage and current
  Series RLC Branch4 : spsSeriesRLCBranchLib/Series RLC Branch  Commented=on  LConnTagsString=__new0  RConnTagsString=__new0  BranchType=C  Resistance=1  Inductance=14e-6  SetiL0=off  InitialCurrent=0  Capacitance=10e-6*(1.25^2)  Setx0=off  InitialVoltage=0  Measurements=Branch voltage and current
  Series RLC Branch5 : spsSeriesRLCBranchLib/Series RLC Branch  Commented=on  LConnTagsString=__new0  RConnTagsString=__new0  BranchType=C  Resistance=1  Inductance=14e-6  SetiL0=off  InitialCurrent=0  Capacitance=10e-6  Setx0=off  InitialVoltage=0  Measurements=Branch voltage and current
  Subsystem3 : Subsystem  Commented=on
  Subsystem4 : Subsystem  Commented=on
  sigmoid : MATLAB Function  Commented=on  TreatAsAtomicUnit=on
  Out1 : Outport
  Out2 : Outport  Port=2
  Out3 : Outport  Port=3
  wires:
  Subsystem3/1(Out1) -> Subsystem4/2(In2)
  From25/1 -> Subsystem4/1(In1)
  From24/1 -> Subsystem3/1(In1)
  In1/1 -> Subsystem3/2(In2)
  Subsystem4/2(Out2) -> Out2/1
  Subsystem4/1(Out1) -> Out1/1
  Subsystem3/2(Out2) -> Out3/1

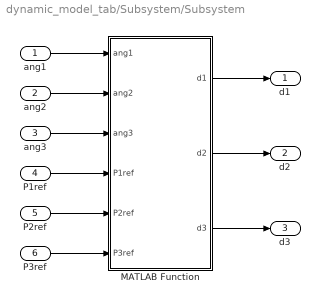
== system dynamic_model_tab/Subsystem/Subsystem ==
  ang1 : Inport
  ang2 : Inport  Port=2
  ang3 : Inport  Port=3
  P1ref : Inport  Port=4
  P2ref : Inport  Port=5
  P3ref : Inport  Port=6
  MATLAB Function : MATLAB Function  TreatAsAtomicUnit=on
  d1 : Outport
  d2 : Outport  Port=2
  d3 : Outport  Port=3
  wires:
  ang1/1 -> MATLAB Function/1(ang1)
  ang2/1 -> MATLAB Function/2(ang2)
  ang3/1 -> MATLAB Function/3(ang3)
  P1ref/1 -> MATLAB Function/4(P1ref)
  P2ref/1 -> MATLAB Function/5(P2ref)
  P3ref/1 -> MATLAB Function/6(P3ref)
  MATLAB Function/1(d1) -> d1/1
  MATLAB Function/2(d2) -> d2/1
  MATLAB Function/3(d3) -> d3/1

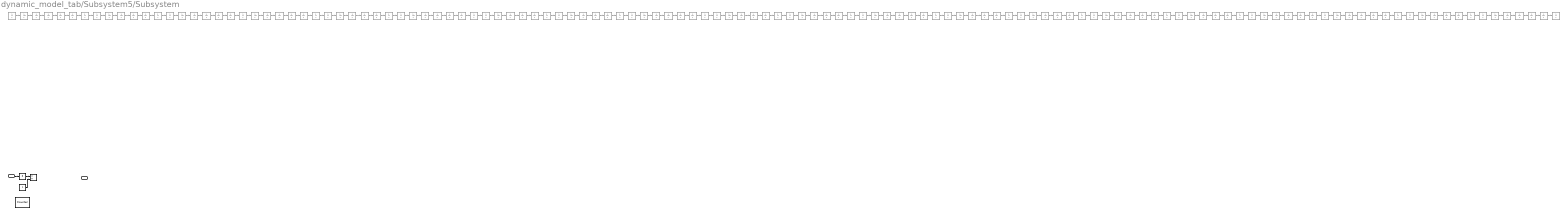
== system dynamic_model_tab/Subsystem5/Subsystem ==
  In1 : Inport
  Constant : Constant
  Counter : eeGeneralControl/Counter  CarrCount=Up  Range=[0 1]  Tper=0.001  Tdelay=0  Ts=0.0001
      settings: LibrarySourceBlock=ee_sl_lib/General Control/Counter
  Divide : Product  Inputs=*/
  Sum of Elements : Sum  Inputs=+  AccumDataTypeStr=int16  SaturateOnIntegerOverflow=on
  Unit Delay{,1..127} (128 alike) : UnitDelay  Commented=on  SampleTime=-1  HasFrameUpgradeWarning=on
  Out1 : Outport
  wires:
  In1/1 -> Sum of Elements/1
  Unit Delay65/1 -> Unit Delay120/1
  Unit Delay126/1 -> Unit Delay127/1
  Unit Delay2/1 -> Unit Delay3/1
  Unit Delay64/1 -> Unit Delay65/1
  Unit Delay125/1 -> Unit Delay98/1
  Unit Delay/1 -> Unit Delay1/1
  Unit Delay82/1 -> Unit Delay72/1
  Unit Delay75/1 -> Unit Delay88/1
  Unit Delay88/1 -> Unit Delay89/1
  Unit Delay72/1 -> Unit Delay73/1
  Unit Delay86/1 -> Unit Delay83/1
  Unit Delay40/1 -> Unit Delay41/1
  Unit Delay17/1 -> Unit Delay28/1
  Unit Delay69/1 -> Unit Delay81/1
  Unit Delay116/1 -> Unit Delay117/1
  Unit Delay87/1 -> Unit Delay64/1
  Unit Delay10/1 -> Unit Delay11/1
  Unit Delay96/1 -> Unit Delay97/1
  Unit Delay78/1 -> Unit Delay103/1
  Unit Delay115/1 -> Unit Delay90/1
  Unit Delay46/1 -> Unit Delay76/1
  Unit Delay77/1 -> Unit Delay78/1
  Unit Delay90/1 -> Unit Delay91/1
  Unit Delay98/1 -> Unit Delay109/1
  Unit Delay26/1 -> Unit Delay27/1
  Unit Delay100/1 -> Unit Delay113/1
  Unit Delay68/1 -> Unit Delay69/1
  Unit Delay120/1 -> Unit Delay125/1
  Unit Delay12/1 -> Unit Delay13/1
  Unit Delay112/1 -> Unit Delay101/1
  Unit Delay50/1 -> Unit Delay40/1
  Unit Delay103/1 -> Unit Delay115/1
  Unit Delay80/1 -> Unit Delay77/1
  Unit Delay124/1 -> Unit Delay96/1
  Unit Delay38/1 -> Unit Delay39/1
  Unit Delay84/1 -> Unit Delay74/1
  Unit Delay73/1 -> Unit Delay85/1
  Unit Delay56/1 -> Unit Delay57/1
  Unit Delay118/1 -> Unit Delay119/1
  Unit Delay89/1 -> Unit Delay79/1
  Unit Delay44/1 -> Unit Delay55/1
  Unit Delay94/1 -> Unit Delay95/1
  Unit Delay43/1 -> Unit Delay56/1
  Unit Delay81/1 -> Unit Delay82/1
  Unit Delay79/1 -> Unit Delay80/1
  Unit Delay58/1 -> Unit Delay59/1
  Unit Delay24/1 -> Unit Delay25/1
  Unit Delay85/1 -> Unit Delay86/1
  Unit Delay97/1 -> Unit Delay94/1
  Unit Delay104/1 -> Unit Delay105/1
  Unit Delay71/1 -> Unit Delay68/1
  Unit Delay127/1 -> Unit Delay70/1
  Unit Delay76/1 -> Unit Delay87/1
  Unit Delay7/1 -> Unit Delay4/1
  Unit Delay108/1 -> Unit Delay110/1
  Unit Delay110/1 -> Unit Delay99/1
  Unit Delay107/1 -> Unit Delay104/1
  Unit Delay117/1 -> Unit Delay106/1
  Unit Delay54/1 -> Unit Delay51/1
  Unit Delay61/1 -> Unit Delay58/1
  Unit Delay122/1 -> Unit Delay118/1
  Unit Delay93/1 -> Unit Delay123/1
  Unit Delay59/1 -> Unit Delay34/1
  Unit Delay51/1 -> Unit Delay52/1
  Unit Delay114/1 -> Unit Delay111/1
  Unit Delay95/1 -> Unit Delay108/1
  Unit Delay83/1 -> Unit Delay84/1
  Unit Delay106/1 -> Unit Delay107/1
  Unit Delay13/1 -> Unit Delay24/1
  Unit Delay113/1 -> Unit Delay114/1
  Unit Delay91/1 -> Unit Delay121/1
  Unit Delay25/1 -> Unit Delay16/1
  Unit Delay121/1 -> Unit Delay122/1
  Unit Delay66/1 -> Unit Delay67/1
  Unit Delay29/1 -> Unit Delay26/1
  Unit Delay101/1 -> Unit Delay102/1
  Unit Delay111/1 -> Unit Delay112/1
  Unit Delay30/1 -> Unit Delay31/1
  Unit Delay70/1 -> Unit Delay71/1
  Unit Delay119/1 -> Unit Delay92/1
  Unit Delay18/1 -> Unit Delay19/1
  Unit Delay67/1 -> Unit Delay126/1
  Unit Delay74/1 -> Unit Delay75/1
  Unit Delay28/1 -> Unit Delay29/1
  Unit Delay102/1 -> Unit Delay116/1
  Unit Delay6/1 -> Unit Delay7/1
  Unit Delay31/1 -> Unit Delay22/1
  Unit Delay63/1 -> Unit Delay38/1
  Unit Delay16/1 -> Unit Delay17/1
  Unit Delay19/1 -> Unit Delay30/1
  Unit Delay22/1 -> Unit Delay23/1
  Unit Delay20/1 -> Unit Delay21/1
  Unit Delay62/1 -> Unit Delay63/1
  Unit Delay32/1 -> Unit Delay33/1
  Unit Delay39/1 -> Unit Delay36/1
  Unit Delay35/1 -> Unit Delay62/1
  Unit Delay37/1 -> Unit Delay49/1
  Unit Delay33/1 -> Unit Delay60/1
  Unit Delay3/1 -> Unit Delay/1
  Unit Delay21/1 -> Unit Delay44/1
  Unit Delay47/1 -> Unit Delay48/1
  Unit Delay42/1 -> Unit Delay43/1
  Unit Delay60/1 -> Unit Delay61/1
  Unit Delay41/1 -> Unit Delay53/1
  Unit Delay23/1 -> Unit Delay20/1
  Unit Delay55/1 -> Unit Delay32/1
  Unit Delay34/1 -> Unit Delay35/1
  Unit Delay11/1 -> Unit Delay8/1
  Unit Delay15/1 -> Unit Delay12/1
  Unit Delay14/1 -> Unit Delay15/1
  Unit Delay53/1 -> Unit Delay54/1
  Unit Delay99/1 -> Unit Delay100/1
  Unit Delay49/1 -> Unit Delay50/1
  Unit Delay45/1 -> Unit Delay46/1
  Unit Delay9/1 -> Unit Delay14/1
  Unit Delay36/1 -> Unit Delay37/1
  Unit Delay123/1 -> Unit Delay124/1
  Unit Delay109/1 -> Unit Delay66/1
  Unit Delay92/1 -> Unit Delay93/1
  Unit Delay5/1 -> Unit Delay10/1
  Unit Delay48/1 -> Unit Delay45/1
  Unit Delay57/1 -> Unit Delay47/1
  Unit Delay52/1 -> Unit Delay42/1
  Unit Delay27/1 -> Unit Delay18/1
  Unit Delay4/1 -> Unit Delay5/1
  Unit Delay8/1 -> Unit Delay9/1
  Unit Delay1/1 -> Unit Delay6/1
  Sum of Elements/1 -> Divide/1
  Constant/1 -> Divide/2

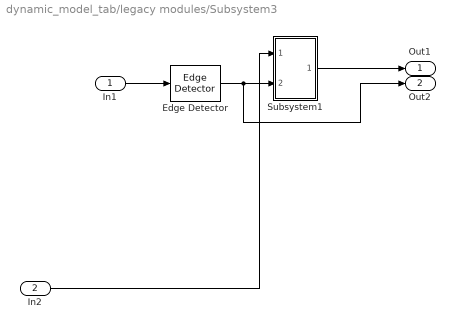
== system dynamic_model_tab/legacy modules/Subsystem3 ==
  In1 : Inport
  In2 : Inport  Port=2
  Edge Detector : spsEdgeDetectorLib/Edge Detector  model=Either  ic=0  Ts=0
      settings: LibrarySourceBlock=sps_lib/Control/Edge Detector
  Subsystem1 : Subsystem
  Out1 : Outport
  Out2 : Outport  Port=2
  wires:
  Edge Detector/1 -> Out2/1, Subsystem1/2(Input)
  Subsystem1/1(Out1) -> Out1/1
  In1/1 -> Edge Detector/1
  In2/1 -> Subsystem1/1(In1)

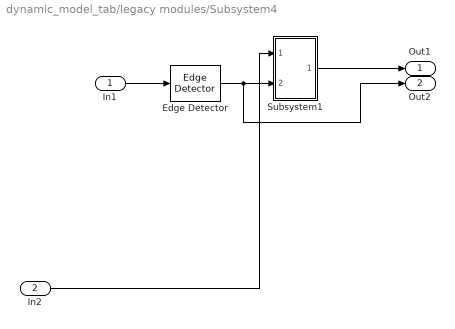
== system dynamic_model_tab/legacy modules/Subsystem4 ==
  In1 : Inport
  In2 : Inport  Port=2
  Edge Detector : spsEdgeDetectorLib/Edge Detector  model=Either  ic=0  Ts=0
      settings: LibrarySourceBlock=sps_lib/Control/Edge Detector
  Subsystem1 : Subsystem
  Out1 : Outport
  Out2 : Outport  Port=2
  wires:
  Edge Detector/1 -> Out2/1, Subsystem1/2(Input)
  Subsystem1/1(Out1) -> Out1/1
  In1/1 -> Edge Detector/1
  In2/1 -> Subsystem1/1(In1)

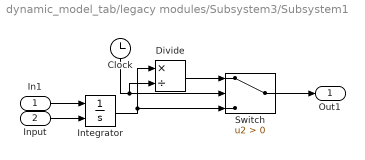
== system dynamic_model_tab/legacy modules/Subsystem3/Subsystem1 ==
  In1 : Inport
  Input : Inport  Port=2
  Clock : Clock
  Divide : Product  Inputs=*/
  Integrator : Integrator  ExternalReset=rising  LimitOutput=on  IgnoreLimit=on
  Switch : Switch  Criteria=u2 > Threshold  SaturateOnIntegerOverflow=off  InputSameDT=off
  Out1 : Outport
  wires:
  Divide/1 -> Switch/1
  Integrator/1 -> Switch/3, Divide/1
  Clock/1 -> Switch/2, Divide/2
  In1/1 -> Integrator/1
  Switch/1 -> Out1/1
  Input/1 -> Integrator/2

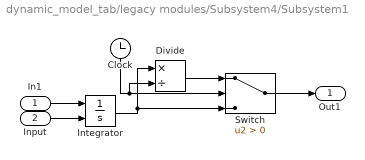
== system dynamic_model_tab/legacy modules/Subsystem4/Subsystem1 ==
  In1 : Inport
  Input : Inport  Port=2
  Clock : Clock
  Divide : Product  Inputs=*/
  Integrator : Integrator  ExternalReset=rising  LimitOutput=on  IgnoreLimit=on
  Switch : Switch  Criteria=u2 > Threshold  SaturateOnIntegerOverflow=off  InputSameDT=off
  Out1 : Outport
  wires:
  Divide/1 -> Switch/1
  Integrator/1 -> Switch/3, Divide/1
  Clock/1 -> Switch/2, Divide/2
  In1/1 -> Integrator/1
  Switch/1 -> Out1/1
  Input/1 -> Integrator/2

== matlab function dynamic_model_tab/Subsystem/SPS ==
  data: u input; pos output; neg output
function [pos,neg] = fcn(u)

if u>=0
    pos = abs(u);
    neg = 0;
else
    neg = abs(u);
    pos = 0;
end

== matlab function dynamic_model_tab/legacy modules/sigmoid ==
  data: u input; y output
function y = fcn(u)

y = 1/(1 + exp(-u));

== matlab function dynamic_model_tab/MATLAB Function ==
  data: p1 input; eff output; p2 input; p3 input
function eff = fcn(p1,p2,p3)

eff = 100*(1-abs(p1+p2+p3)/max(abs(p1),max(abs(p2),abs(p3))));

== matlab function dynamic_model_tab/Subsystem/Subsystem/MATLAB Function ==
  data: ang1 input; d1 output; ang2 input; ang3 input; d2 output; d3 output; P1ref input; P2ref input; P3ref input
function [d1,d2,d3] = fcn(ang1, ang2, ang3, P1ref, P2ref, P3ref)
[~, i] = max([P1ref,P2ref,P3ref]);

d1 = ang1;
d2 = ang2;
d3 = ang3;

% if i==1
%     d1 = 0;
%     d2 = ang2;
%     d3 = ang3;
% elseif i==2
%     d1 = ang1;
%     d2 = 0;
%     d3 = ang3;
% else
%     d1 = ang1;
%     d2 = ang2;
%     d3 = 0;
% end

== matlab function dynamic_model_tab/MATLAB Function1 ==
  data: pref1 input; Prefout1 output; pref2 input; pref3 input; Prefout2 output; Prefout3 output
function [Prefout1, Prefout2, Prefout3]= fcn(pref1, pref2, pref3)
P = [pref1,pref2,pref3];

[~,i] = max(isnan(P));

if i==1
    Prefout1 = -1*sum(P,'omitnan');
    Prefout2 = pref2;
    Prefout3 = pref3;
elseif i==2
    Prefout2 = -1*sum(P,'omitnan');
    Prefout1 = pref1;
    Prefout3 = pref3;
elseif i == 3
    Prefout3 = -1*sum(P,'omitnan');
    Prefout2 = pref2;
    Prefout1 = pref1;
else
    Prefout1 = pref1;
    Prefout2 = pref2;
    Prefout3 = pref3;
end
